simulink model "compTF"  (Simulink 6.4)
settings: Solver=ode4  StartTime=0.0  StopTime=cas_simulacie  FixedStep=ptv_sim_step  RelTol=1e-3
values from neighbouring files (symbols this model uses):
  DD2 = D_km;end,naspat_porovn=''close,id_param'';porovnat')    [id_param.m]
  K = get(findobj('Tag','ptt_s4'),'Value')    [id_tune.m]    (also in id_tune_pe_zal.m = id_backup(2); id_tune_zal.m = y_norm(end); km_id.m = 0; km_sustavy.m = y_nek)
  M = (y_max-y_min)/y_max    [km_id.m]    (also in km_sustavy.m)
undefined symbols (not defined in the file or in its folder): DD, L, N
settings Model: Creator=oravec  LastModifiedBy=oravec
settings DataIOCC: LimitDataPoints=off  SignalLoggingName=sigsOut
settings OptimizationCC: InitFltsAndDblsToZero=off
settings DebuggingCC: SolverPrmCheckMsg=none  StrictBusMsg=None
settings HardwareCC: TargetHWDeviceType=32-bit Generic  TargetUnknown=on  ProdEqTarget=off

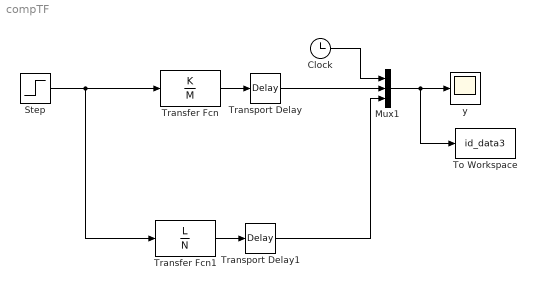
== system compTF ==
  Clock : Clock
      settings: Decimation=10
  Mux1 : Mux  Inputs=3
  Step : Step  Time=0  SampleTime=0
  To Workspace : ToWorkspace  VariableName=id_data3  SampleTime=-1  SaveFormat=Array
  Transfer Fcn : TransferFcn  Numerator=K  Denominator=M
  Transfer Fcn1 : TransferFcn  Numerator=L  Denominator=N
  Transport Delay : TransportDelay  DelayTime=DD2
  Transport Delay1 : TransportDelay  DelayTime=DD
  y : Scope
      settings: SaveName=ScopeData2
  wires:
  Step/1 -> Transfer Fcn/1, Transfer Fcn1/1
  Transfer Fcn/1 -> Transport Delay/1
  Transport Delay/1 -> Mux1/2
  Clock/1 -> Mux1/1
  Mux1/1 -> y/1, To Workspace/1
  Transfer Fcn1/1 -> Transport Delay1/1
  Transport Delay1/1 -> Mux1/3
